simulink model "slb_seri_para"  (R2015b)
settings: Solver=FixedStepDiscrete  SolverMode=SingleTasking  StartTime=0.0  StopTime=2  RelTol=1e-3
libraries: simulink x2, hdlsllib x1, dspindex x1
settings Model: DataTypeOverride=Off  Creator=amatsumo  LastModifiedBy=amatsumo
settings DataIOCC: SaveFormat=Array  SaveOutput=off  SignalLogging=off  SaveTime=off
settings OptimizationCC: BlockReduction=off  ConditionallyExecuteInputs=off  DefaultParameterBehavior=Inlined
settings DebuggingCC: AlgebraicLoopMsg=error  UnderspecifiedInitializationDetection=Classic  MergeDetectMultiDrivingBlocksExec=none  SolverPrmCheckMsg=warning  SingleTaskRateTransMsg=error  StateNameClashWarn=warning
settings HardwareCC: ProdBitPerPointer=32  ProdLargestAtomicFloat=None  ProdIntDivRoundTo=Undefined  ProdEndianess=Unspecified  ProdWordSize=32  ProdHWDeviceType=ASIC/FPGA->ASIC/FPGA  ProdEqTarget=off
settings GRTTargetCC: GeneratePreprocessorConditionals=Disable all
settings ConfigComp: CovModelRefEnable=Off  CovSFcnEnable=off

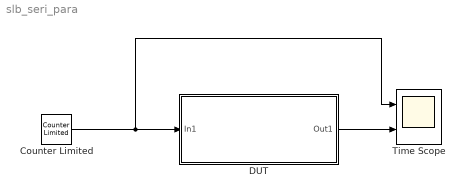
== system slb_seri_para ==
  Counter Limited : simulink/Sources/Counter Limited  uplimit=32  tsamp=1/100
  DUT : Subsystem
  Time Scope : Scope  NumInputPorts=2
  wires:
  Counter Limited/1 -> DUT/1(In1), Time Scope/1
  DUT/1(Out1) -> Time Scope/2

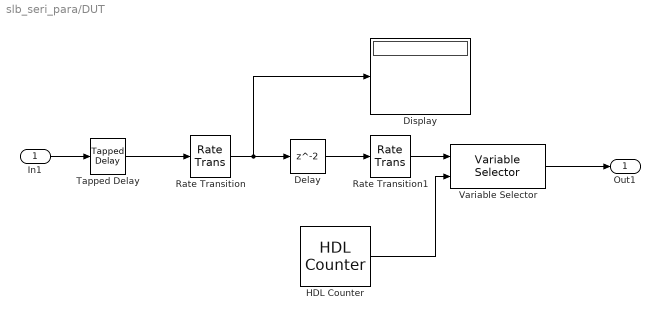
== system slb_seri_para/DUT ==
  In1 : Inport
  Delay : Delay
  Display : Display
  HDL Counter : hdlsllib/HDL Operations/HDL Counter  CountType=Count limited  CountInit=0  CountStep=1  CountMax=15  CountFromType=Initial value  CountFrom=0  CountResetPort=off  CountLoadPort=off  CountEnbPort=off  CountDirPort=off  CountDataType=Unsigned  CountWordLen=8  CountFracLen=0  CountSampTime=-1
  Rate Transition : RateTransition  OutPortSampleTimeOpt=Multiple of input port sample time  OutPortSampleTimeMultiple=16
  Rate Transition1 : RateTransition  OutPortSampleTimeOpt=Multiple of input port sample time  OutPortSampleTimeMultiple=1/16
  Tapped Delay : simulink/Discrete/Tapped Delay  vinit=0.0  samptime=-1  NumDelays=15  DelayOrder=Oldest  includeCurrent=on
  Variable Selector : dspindex/Variable Selector  NumInputs=1  rowsOrCols=Rows  IdxMode=Variable  Elements=[1 3]  ZerOneIdxMode=Zero-based  errmode=Clip Index  FillMode=on  FillValues=0
  Out1 : Outport
  wires:
  Delay/1 -> Rate Transition1/1
  Rate Transition/1 -> Display/1, Delay/1
  Tapped Delay/1 -> Rate Transition/1
  Variable Selector/1 -> Out1/1
  Rate Transition1/1 -> Variable Selector/1
  HDL Counter/1 -> Variable Selector/2
  In1/1 -> Tapped Delay/1
